simulink model "filtr_kalmana"  (R2022b)
settings: Solver=ode3  StartTime=0.0  StopTime=0.35  FixedStep=Tp  RelTol=1e-3
values from neighbouring files (symbols this model uses):
  a21 = 1/2/m * x30^2 * FemP1/FemP2^2 * exp(-x10/FemP2)    [init.m]    (also in proj.m)
  a23 = -1/m * x30 * FemP1/FemP2 * exp(-x10/FemP2)    [init.m]    (also in proj.m)
  a31 = 1/f1 * exp(x10/f2) * (ki*u10 + ci - x30)    [init.m]    (also in proj.m)
  a33 = -f2/f1 * exp(x10/f2)    [init.m]    (also in proj.m)
  Ad = eye(3) + A*Tp    [init.m]
  b31 = ki * f2/f1 * exp(x10/f2)    [init.m]    (also in proj.m)
  Bd = B(:,1)*Tp    [init.m]
  Cd = C    [init.m]
  g = 9.81    [init.m]    (also in proj.m)
  K = place(A, B(:, 1), [-28, -60, -90])    [init.m]    (also in proj.m)
  xd = d-bd    [init.m]    (also in proj.m)
settings Model: Creator=minekuba  LastModifiedBy=minekuba

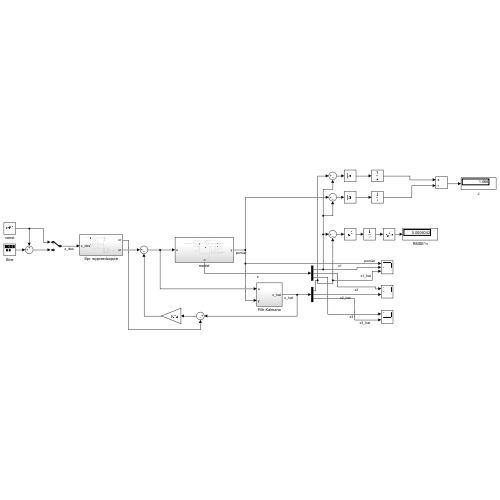
[thumbnail: Simulink's stored preview of the top-level diagram]
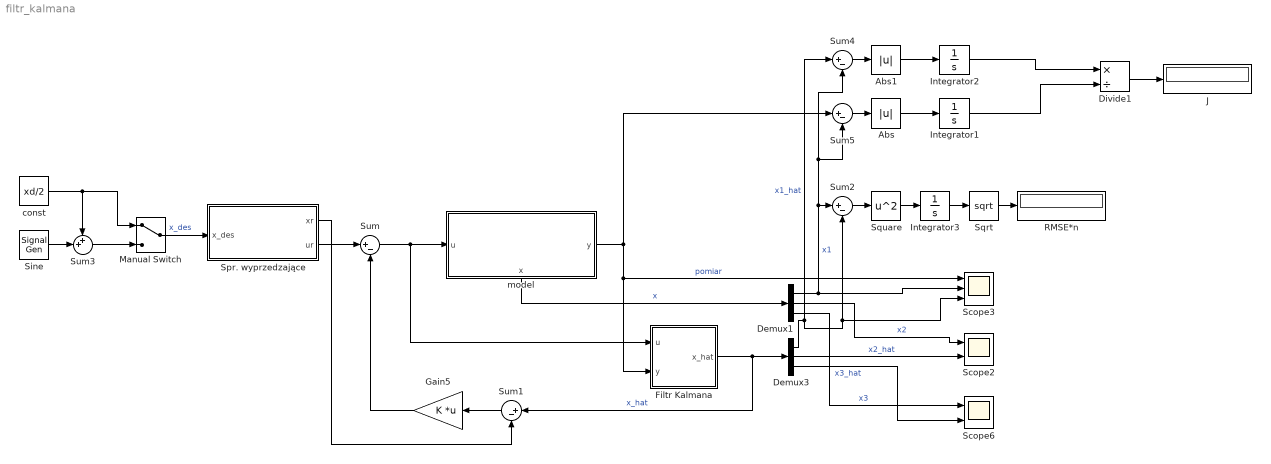
== system filtr_kalmana ==
  Abs : Abs  SaturateOnIntegerOverflow=off
  Abs1 : Abs  SaturateOnIntegerOverflow=off
  Demux1 : Demux  Outputs=3
  Demux3 : Demux  Outputs=3
  Divide1 : Product  Inputs=*/
  Filtr Kalmana : Subsystem
  Gain5 : Gain  Gain=K  Multiplication=Matrix(K*u)
  Integrator1 : Integrator
  Integrator2 : Integrator
  Integrator3 : Integrator
  J : Display
  Manual Switch : ManualSwitch
  RMSE*n : Display
  Scope2 : Scope  NumInputPorts=2
  Scope3 : Scope  NumInputPorts=3
  Scope6 : Scope  NumInputPorts=2
  Sine : SignalGenerator  Amplitude=xd/12  Frequency=0.2
  Spr. wyprzedzające : Subsystem
  Sqrt : Sqrt
  Square : Math  Operator=square
  Sum{,1..2,4..5} (5 alike) : Sum  Inputs=|+-
  Sum3 : Sum  Inputs=++|
  const : Constant  Value=xd/2
  model : Subsystem
      settings: PortSchema="{\"entries\":[{\"content\":{\"sides\":[{\"content\":{\"connectorIds\":[\"In1\"]},\"type\":\"ConnectorPlacement.EquallySpacedRectSide\",\"uuid\":\"08100310-f669-4bec-b75a-4c341ab1329c\"},{\"content\":{\"connectorIds\":[\"Out1\"],\"side\":\"RIGHT\"},\"type\":\"ConnectorPlacement.EquallySpacedRectSide\",\"uuid\":\"75a75395-bc88-4968-acfb-02365cdbbaac\"},{\"content\":{\"connectorIds\":[],\"side\":\"TOP\"},\"type\":\"ConnectorPlacement.EquallySpacedRectSide\",\"uuid\":\"7e90434d-1931-47ff-b270-f1d54f71bb7e\"},{\"content\":{\"connectorIds\":[\"Out2\"],\"side\":\"BOTTOM\"},\"type\":\"ConnectorPlacement.EquallySpacedRectSide\",\"uuid\":\"09ce4af7-043c-4542-961c-50c1fb378fc1\"}]},\"type\":\"ConnectorPlacement.EquallySpacedConnector\",\"uuid\":\"9c93e3e1-5fb5-4a02-9a28-f46059e1f065\"}],\"packageUris\":[\"http://schema.mathworks.com/mf0/Connector/R2020b\"],\"version\":\"1.0\"}"
  wires:
  Sum/1 -> Filtr Kalmana/1(u), model/1(u)
  Sum1/1 -> Gain5/1
  Sine/1 -> Sum3/2
  Gain5/1 -> Sum/2
  Spr. wyprzedzające/2(ur) -> Sum/1
  const/1 -> Sum3/1, Manual Switch/1
  Spr. wyprzedzające/1(xr) -> Sum1/2
  Sum3/1 -> Manual Switch/2
  model/1(y) -> Scope3/1, Filtr Kalmana/2(y), Sum5/1  "pomiar"
  Manual Switch/1 -> Spr. wyprzedzające/1(x_des)  "x_des"
  Filtr Kalmana/1(x_hat) -> Sum1/1, Demux3/1  "x_hat"
  Demux1/2 -> Scope2/1  "x2"
  Demux3/1 -> Sum4/1, Scope3/3, Sum2/2  "x1_hat"
  Demux3/2 -> Scope2/2  "x2_hat"
  Demux3/3 -> Scope6/2  "x3_hat"
  Demux1/3 -> Scope6/1  "x3"
  Demux1/1 -> Scope3/2, Sum4/2, Sum5/2, Sum2/1  "x1"
  model/2(x) -> Demux1/1  "x"
  Sum2/1 -> Square/1
  Sqrt/1 -> RMSE*n/1
  Square/1 -> Integrator3/1
  Integrator3/1 -> Sqrt/1
  Sum5/1 -> Abs/1
  Sum4/1 -> Abs1/1
  Abs1/1 -> Integrator2/1
  Abs/1 -> Integrator1/1
  Integrator1/1 -> Divide1/2
  Integrator2/1 -> Divide1/1
  Divide1/1 -> J/1

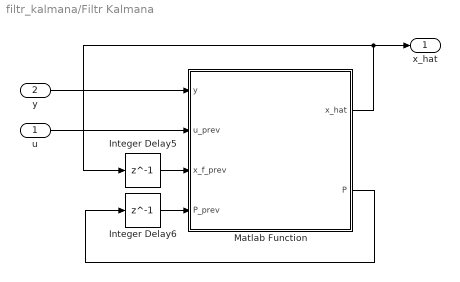
== system filtr_kalmana/Filtr Kalmana ==
  u : Inport
  y : Inport  Port=2
  Integer Delay5 : Delay  DelayLength=1  InitialCondition=[0.0105; 0; 0]
  Integer Delay6 : Delay  DelayLength=1  InitialCondition=eye(3)
  Matlab Function : MATLAB Function  TreatAsAtomicUnit=on
  x_hat : Outport
  wires:
  y/1 -> Matlab Function/1(y)
  Matlab Function/1(x_hat) -> x_hat/1, Integer Delay5/1
  u/1 -> Matlab Function/2(u_prev)
  Matlab Function/2(P) -> Integer Delay6/1
  Integer Delay6/1 -> Matlab Function/4(P_prev)
  Integer Delay5/1 -> Matlab Function/3(x_f_prev)

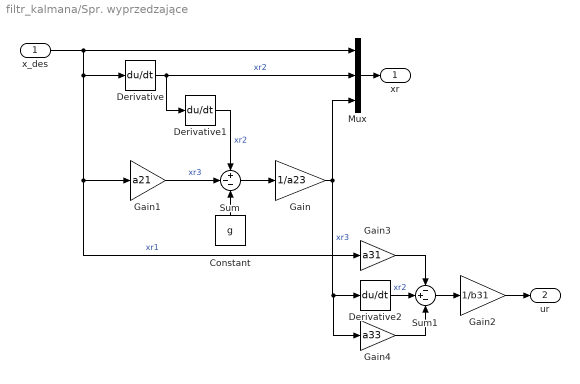
== system filtr_kalmana/Spr. wyprzedzające ==
  x_des : Inport
  Constant : Constant  Value=g
  Derivative : Derivative
  Derivative1 : Derivative
  Derivative2 : Derivative
  Gain : Gain  Gain=1/a23
  Gain1 : Gain  Gain=a21
  Gain2 : Gain  Gain=1/b31
  Gain3 : Gain  Gain=a31
  Gain4 : Gain  Gain=a33
  Mux : Mux  Inputs=3
  Sum : Sum  Inputs=+--
  Sum1 : Sum  Inputs=-+-
  xr : Outport
  ur : Outport  Port=2
  wires:
  Mux/1 -> xr/1
  x_des/1 -> Gain3/1, Gain1/1, Derivative/1, Mux/1  "xr1"
  Derivative/1 -> Derivative1/1, Mux/2  "xr2"
  Gain/1 -> Gain4/1, Derivative2/1, Mux/3  "xr3"
  Derivative1/1 -> Sum/1  "xr2"
  Sum/1 -> Gain/1
  Constant/1 -> Sum/3
  Gain1/1 -> Sum/2  "xr3"
  Gain2/1 -> ur/1
  Sum1/1 -> Gain2/1
  Derivative2/1 -> Sum1/2  "xr2"
  Gain3/1 -> Sum1/1
  Gain4/1 -> Sum1/3

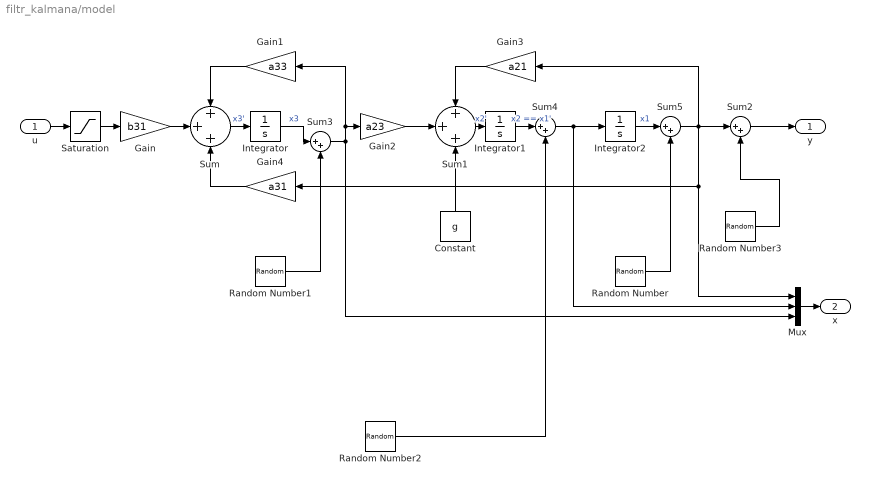
== system filtr_kalmana/model ==
  u : Inport
  Constant : Constant  Value=g
  Gain : Gain  Gain=b31
  Gain1 : Gain  Gain=a33
  Gain2 : Gain  Gain=a23
  Gain3 : Gain  Gain=a21
  Gain4 : Gain  Gain=a31
  Integrator : Integrator
  Integrator1 : Integrator
  Integrator2 : Integrator  InitialCondition=xd  LimitOutput=on  UpperSaturationLimit=xd  LowerSaturationLimit=0
  Mux : Mux  Inputs=3
  Random Number : RandomNumber  Variance=0.0000001  Seed=2137  SampleTime=0.001
  Random Number1 : RandomNumber  Variance=0.00001  Seed=123  SampleTime=0.0001
  Random Number2 : RandomNumber  Variance=0.00001  Seed=420  SampleTime=0.001
  Random Number3 : RandomNumber  Variance=0.000001  Seed=2137  SampleTime=0.0001
  Saturation : Saturate  UpperLimit=1  LowerLimit=0
  Sum : Sum  Inputs=+++
  Sum1 : Sum  Inputs=+++
  Sum{2..5} (4 alike) : Sum  Inputs=|++
  y : Outport
  x : Outport  Port=2
  wires:
  Gain1/1 -> Sum/1
  Integrator/1 -> Sum3/1  "x3"
  Constant/1 -> Sum1/3
  Gain/1 -> Sum/2
  Gain4/1 -> Sum/3
  u/1 -> Saturation/1
  Sum/1 -> Integrator/1  "x3'"
  Gain3/1 -> Sum1/1
  Sum1/1 -> Integrator1/1  "x2'"
  Saturation/1 -> Gain/1
  Gain2/1 -> Sum1/2
  Mux/1 -> x/1
  Random Number/1 -> Sum5/2
  Sum3/1 -> Gain1/1, Gain2/1, Mux/3
  Random Number1/1 -> Sum3/2
  Integrator1/1 -> Sum4/1  "x2 == x1'"
  Sum4/1 -> Mux/2, Integrator2/1
  Random Number2/1 -> Sum4/2
  Integrator2/1 -> Sum5/1  "x1"
  Sum2/1 -> y/1
  Sum5/1 -> Sum2/1, Gain4/1, Mux/1, Gain3/1
  Random Number3/1 -> Sum2/2

== matlab function filtr_kalmana/Filtr Kalmana/Matlab Function ==
  settings: sampleTime=0.0005
  settings: fimath=|
      | fimath(...
      | 'RoundMode', 'floor',...
      | 'OverflowMode', 'wrap',...
      | 'ProductMode', 'KeepLSB', 'ProductWordLength', 32,...
      | 'SumMode', 'KeepLSB', 'SumWordLength', 32,...
      | 'CastBeforeSum', false)
  data: y input; u_prev input; x_hat output; x_f_prev input; P_prev input; P output; Ad parameter double; Cd parameter double; Bd parameter double
function [x_hat, P] = kalman_filter(y, u_prev, x_f_prev, P_prev, Ad, Cd, Bd)
Q = diag([0.0000012 0.05 0.0001]);
R = 3;

x_pred = Ad*x_f_prev + Bd*u_prev;
P_pred = Ad*P_prev*Ad' + Q;

K = P_pred * Cd' * (Cd*P_pred*Cd' + R)^-1;
x_f = x_pred + K * (y - x_pred(1));

P = (eye(3) - K * Cd) * P_pred;
x_hat = x_f;
